simulink model "safecomp_demo"  (R2024a)
settings: Solver=VariableStepAuto  StartTime=0.0  StopTime=10.0  RelTol=1e-3
undefined symbols (not defined in the file): Defined, Ego, Lane, User
libraries: roadrunnerscenario x2
settings Model: Creator=matsulab  LastModifiedBy=matsulab

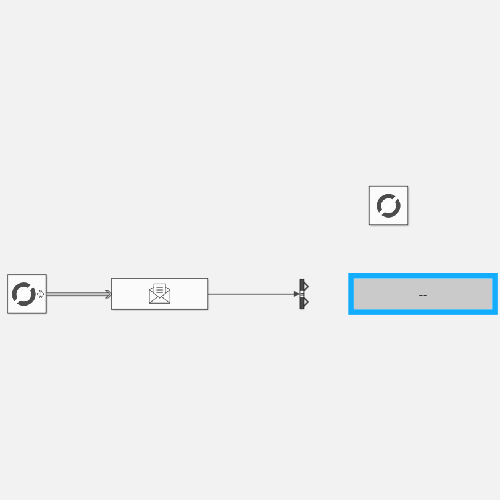
[thumbnail: Simulink's stored preview of the top-level diagram]
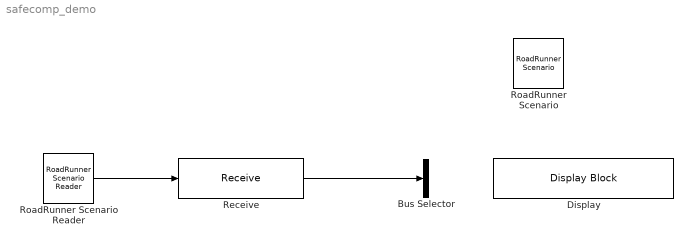
== system safecomp_demo ==
  Bus Selector : BusSelector  OutputSignals=signal1,signal2
  Display : DisplayBlock  LabelPosition=Hide  Transparency=1
  Receive : Receive  InputPortMessageModes=m  UseInternalQueue=off  QueueOverwriting=on  QueueLength=1  QueueType=LIFO
  RoadRunner Scenario : roadrunnerscenario/RoadRunner Scenario  UserDefinedActions={}  UserDefinedEvents={}
  RoadRunner Scenario Reader : roadrunnerscenario/RoadRunner Scenario Reader  TopicCategory=Action  ActorCategory=All Types  ActionType=Speed Change  EventType=User-Defined  TopicType=Actor Specifications  VehicleType=Vehicle Specifications  UserDefinedAction=Action1  UserDefinedEvent=Event1  Filter=Self  SensorTopic=Target Poses  LaneBoundaryOutputTopic=Ego-Lane  SensorID=1  SampleTime=0
  wires:
  RoadRunner Scenario Reader/1 -> Receive/1
  Receive/1 -> Bus Selector/1
